simulink model "Go_continua"  (Simulink 5.0)
settings: Solver=ode45  StartTime=0.0  StopTime=10.0  RelTol=1e-3
undefined symbols (not defined in the file): q, Vd, Vm
settings Model: LastModifiedBy=pc1

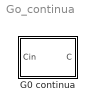
== system Go_continua ==
  G0 continua : Subsystem

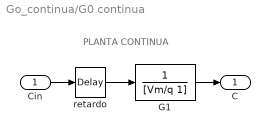
== system Go_continua/G0 continua ==
  note: PLANTA CONTINUA
  Cin : Inport
  G1 : TransferFcn  Denominator=[Vm/q 1]
  retardo : TransportDelay  DelayTime=Vd/q
  C : Outport
  wires:
  retardo/1 -> G1/1
  G1/1 -> C/1
  Cin/1 -> retardo/1
